simulink library "vehicleMotionVisualiser"  (R2024b)
settings: Solver=VariableStepAuto  StartTime=0.0  StopTime=10.0  RelTol=1e-3
libraries: vehdynlibviscommon x1
settings Model: Creator=Josue  LastModifiedBy=Josue

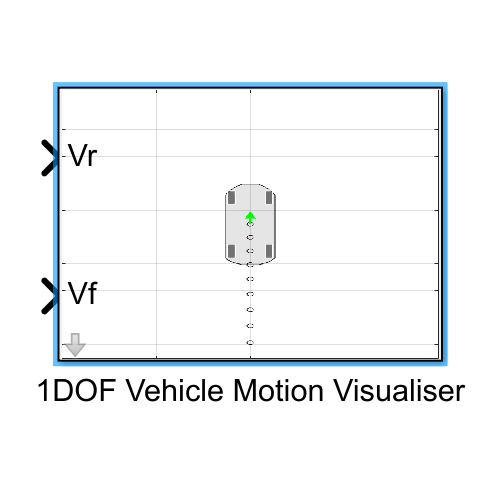
[thumbnail: Simulink's stored preview of the top-level diagram]
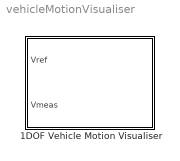
== system vehicleMotionVisualiser ==
  1DOF Vehicle Motion Visualiser : Subsystem
      mask DialogControl DescGroupVar Prompt: 1DOF Vehicle Motion Visualiser
      mask DialogControl DescTextVar Prompt: Provides a 1-degree-of-freedom longitudinal vehicle simulation with integrated XY-plane visualization. This component outputs position, velocity, and reference trajectory data to the Vehicle XY Plotter for real-time motion display.
      mask Display:
      | image('documentation\pictures\vehicleMotionVisualiserMask.PNG');
      | port_label('input', 1, 'Vr');
      | port_label('input', 2, 'Vf');

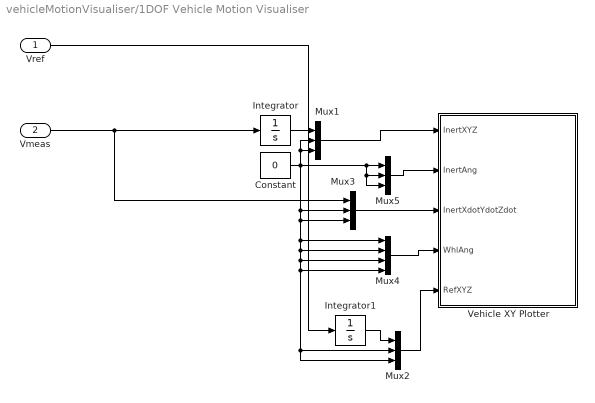
== system vehicleMotionVisualiser/1DOF Vehicle Motion Visualiser ==
  Vref : Inport
  Vmeas : Inport  Port=2
  Constant : Constant  Value=0
  Integrator : Integrator
  Integrator1 : Integrator
  Mux{1..3,5} (4 alike) : Mux  Inputs=3
  Mux4 : Mux
  Vehicle XY Plotter : Subsystem  mask(Vehicle XY Plotter){extRef=on, extStats=off, extTireF=off, a=2, b=2, w=2, figBorder=10, bufferSize=1024, velNorm=5, tireFNorm=1000, pltDT=0.2}
      mask prompts: extRef "Plot path reference, extRef"; extStats "Display speed, RPM and Gear"; extTireF "Display tire forces"; a "Distance to front axle from CG, a [m]:"; b "Distance to rear axle from CG, b [m]:"; w "Track width, w [m]:"; figBorder "Distance to figure borders, figBorder [m]:"; bufferSize "Path buffer sampe size, bufferSize []:"; velNorm "Velocity vector scaling, velNorm [m*s/m]:"; tireFNorm "Tire force vector scaling, tireFNorm [m/N]:"; pltDT "Plot update rate, pltDT [s]:"
      mask help:
      | This block will display a MATLAB figure which indicates the vehicle path, current position and heading velocity.
      | An optional path reference is also provided.
      mask init:
      | % Mask Initialization: Vehicle 1DOF Visualiser
      | % Cleaned version, no internal dependencies
      | 
      | block = gcb;
      | 
      | % Define inport order and ports explicitly (no AutoBlocks logic)
      | InportNames = {'InertXYZ'; 'InertAng'; 'InertXdotYdotZdot'; 'WhlAng'; 'RefXYZ'};
      | 
      | for idx = 1:length(InportNames)
      |     blkPath = [block '/' InportNames{idx}];
      |     if bdIsLoaded(bdroot(block)) && ~isempty(find_system(block, 'SearchDepth', 1, 'Name', InportNames{idx}))
      |         set_param(blkPath, 'Port', num2str(idx));
      |     end
      | end
      mask TypeOptions a: Vehicle XY Plotter/a
      mask TypeOptions b: Vehicle XY Plotter/b
      mask TypeOptions w: Vehicle XY Plotter/w
      mask TypeOptions figBorder: Vehicle XY Plotter/figBorder
      mask TypeOptions bufferSize: Vehicle XY Plotter/bufferSize
      mask TypeOptions velNorm: Vehicle XY Plotter/velNorm
      mask TypeOptions tireFNorm: Vehicle XY Plotter/tireFNorm
      mask DialogControl Container3 Prompt: Plot and Display Options
  wires:
  Constant/1 -> Mux5/3, Mux5/2, Mux5/1, Mux3/2, Mux4/1, Mux4/3, Mux2/3, Mux2/2, Mux4/4, Mux4/2, Mux3/3, Mux1/3, Mux1/2
  Integrator1/1 -> Mux2/1
  Mux2/1 -> Vehicle XY Plotter/5(RefXYZ)
  Integrator/1 -> Mux1/1
  Mux5/1 -> Vehicle XY Plotter/2(InertAng)
  Mux4/1 -> Vehicle XY Plotter/4(WhlAng)
  Mux3/1 -> Vehicle XY Plotter/3(InertXdotYdotZdot)
  Vmeas/1 -> Mux3/1, Integrator/1
  Mux1/1 -> Vehicle XY Plotter/1(InertXYZ)
  Vref/1 -> Integrator1/1

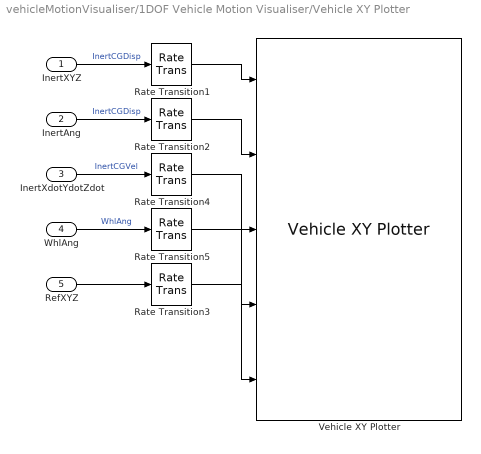
== system vehicleMotionVisualiser/1DOF Vehicle Motion Visualiser/Vehicle XY Plotter ==
  InertXYZ : Inport
  InertAng : Inport  Port=2
  InertXdotYdotZdot : Inport  Port=3
  WhlAng : Inport  Port=4
  RefXYZ : Inport  Port=5
  Rate Transition{1..5} (5 alike) : RateTransition  Deterministic=off  OutPortSampleTime=pltDT
  Vehicle XY Plotter : vehdynlibviscommon/Vehicle XY Plotter  w=w  a=a  b=b  figBorder=figBorder  bufferSize=bufferSize  extStats=off  extTireF=off
  wires:
  RefXYZ/1 -> Rate Transition3/1
  Rate Transition5/1 -> Vehicle XY Plotter/4
  Rate Transition4/1 -> Vehicle XY Plotter/3
  Rate Transition2/1 -> Vehicle XY Plotter/2
  Rate Transition1/1 -> Vehicle XY Plotter/1
  Rate Transition3/1 -> Vehicle XY Plotter/5
  WhlAng/1 -> Rate Transition5/1  "WhlAng"
  InertXYZ/1 -> Rate Transition1/1  "InertCGDisp"
  InertXdotYdotZdot/1 -> Rate Transition4/1  "InertCGVel"
  InertAng/1 -> Rate Transition2/1  "InertCGDisp"
